simulink model "building_EXAMPLE_v1"  (R2016b)
settings: Solver=ode23tb  StartTime=-building.preruntime+8760*3600  StopTime=building.runtime+8760*3600  MaxStep=600  EnableMultiTasking=on
StartFcn:
  | tic
StopFcn:
  | toc
values from neighbouring files (symbols this model uses):
  building = create_building_automatic(building, modify, import_mode, name_XML, name_EXCEL, name_PHPP, NUMBEROFZONES)    [work_EXAMPLE_v1.m]
undefined symbols (not defined in the file or in its folder): A, B, C, cp, Dd, Dreifach, FluidMix, get_building, ID, MassFlow, p, Pressure, Qdot_C, Qdot_C_energy, Qdot_H, Qdot_H_energy, Qdot_I_electricity, Qdot_I_electricity_energy, Qdot_I_light, Qdot_I_light_energy, Qdot_I_person, Qdot_I_person_energy, Qdot_S, Qdot_S_energy, Qdot_T_ground, Qdot_T_ground_energy, Qdot_T_neighbour, Qdot_T_neighbour_energy, Qdot_T_opaque, Qdot_T_opaque_energy, Qdot_T_window, Qdot_T_window_energy, Qdot_V_infiltration, Qdot_V_infiltration_energy, Qdot_V_mech, Qdot_V_mech_energy, Qdot_V_window, Qdot_V_window_energy, rho, Tc, Temperature, Tr, Ts, Wärmeschutzglas, x_CO2, x_H2O, x_VOC
libraries: carnotUIBK x1931, carnot x83, simulink_extras x22, simulink x12
(part 35 of 35)

== system building_EXAMPLE_v1/HVAC pipes/ventilation_pipe_out_1/mix4 ==
  THB_1 : Inport
  THB_2 : Inport  Port=2
  Add{,1..3} (4 alike) : Sum
  Bus Assignment : BusAssignment  AssignedSignals=Temperature,MassFlow,Pressure,FluidMix
  Bus Selector : BusSelector  OutputSignals=Temperature,MassFlow,Pressure,FluidMix
  Bus Selector2 : BusSelector  OutputSignals=Temperature,MassFlow,Pressure,FluidMix
  Divide : Product  Inputs=*/
  Divide1 : Product  Inputs=*/
  Divide2 : Product  Inputs=*/
  Product{,1..5} (6 alike) : Product
  THB : Outport
  wires:
  Add/1 -> Divide/1  "theta"
  Product1/1 -> Add/2
  Product/1 -> Add/1
  THB_1/1 -> Bus Assignment/1, Bus Selector/1
  Add2/1 -> Divide1/1  "p"
  Product2/1 -> Add2/1
  Product3/1 -> Add2/2
  THB_2/1 -> Bus Selector2/1
  Product4/1 -> Add3/1
  Product5/1 -> Add3/2
  Add3/1 -> Divide2/1  "x"
  Add1/1 -> Divide/2, Divide1/2, Divide2/2, Bus Assignment/3  "massflow"
  Bus Assignment/1 -> THB/1
  Divide2/1 -> Bus Assignment/5
  Divide1/1 -> Bus Assignment/4
  Divide/1 -> Bus Assignment/2
  Bus Selector/1 -> Product/1  "<Temperature>"
  Bus Selector2/1 -> Product1/1  "<Temperature>"
  Bus Selector/3 -> Product2/2  "<Pressure>"
  Bus Selector2/3 -> Product3/2  "<Pressure>"
  Bus Selector/4 -> Product4/2  "<FluidMix>"
  Bus Selector2/4 -> Product5/2  "<FluidMix>"
  Bus Selector/2 -> Product4/1, Product2/1, Add1/1, Product/2  "<MassFlow>"
  Bus Selector2/2 -> Add1/2, Product1/2, Product5/1, Product3/1  "<MassFlow>"

== system building_EXAMPLE_v1/HVAC pipes/ventilation_pipe_out_1/mix5 ==
  THB_1 : Inport
  THB_2 : Inport  Port=2
  Add{,1..3} (4 alike) : Sum
  Bus Assignment : BusAssignment  AssignedSignals=Temperature,MassFlow,Pressure,FluidMix
  Bus Selector : BusSelector  OutputSignals=Temperature,MassFlow,Pressure,FluidMix
  Bus Selector2 : BusSelector  OutputSignals=Temperature,MassFlow,Pressure,FluidMix
  Divide : Product  Inputs=*/
  Divide1 : Product  Inputs=*/
  Divide2 : Product  Inputs=*/
  Product{,1..5} (6 alike) : Product
  THB : Outport
  wires:
  Bus Selector2/2 -> Product3/1, Product5/1, Product1/2, Add1/2  "<MassFlow>"
  Bus Selector/2 -> Product/2, Add1/1, Product2/1, Product4/1  "<MassFlow>"
  Bus Selector2/4 -> Product5/2  "<FluidMix>"
  Bus Selector/4 -> Product4/2  "<FluidMix>"
  Bus Selector2/3 -> Product3/2  "<Pressure>"
  Bus Selector/3 -> Product2/2  "<Pressure>"
  Bus Selector2/1 -> Product1/1  "<Temperature>"
  Bus Selector/1 -> Product/1  "<Temperature>"
  Divide/1 -> Bus Assignment/2
  Divide1/1 -> Bus Assignment/4
  Divide2/1 -> Bus Assignment/5
  Bus Assignment/1 -> THB/1
  Add1/1 -> Bus Assignment/3, Divide2/2, Divide1/2, Divide/2  "massflow"
  Add3/1 -> Divide2/1  "x"
  Product5/1 -> Add3/2
  Product4/1 -> Add3/1
  THB_2/1 -> Bus Selector2/1
  Product3/1 -> Add2/2
  Product2/1 -> Add2/1
  Add2/1 -> Divide1/1  "p"
  THB_1/1 -> Bus Selector/1, Bus Assignment/1
  Product/1 -> Add/1
  Product1/1 -> Add/2
  Add/1 -> Divide/1  "theta"

== system building_EXAMPLE_v1/HVAC pipes/ventilation_pipe_out_1/mix6 ==
  THB_1 : Inport
  THB_2 : Inport  Port=2
  Add{,1..3} (4 alike) : Sum
  Bus Assignment : BusAssignment  AssignedSignals=Temperature,MassFlow,Pressure,FluidMix
  Bus Selector : BusSelector  OutputSignals=Temperature,MassFlow,Pressure,FluidMix
  Bus Selector2 : BusSelector  OutputSignals=Temperature,MassFlow,Pressure,FluidMix
  Divide : Product  Inputs=*/
  Divide1 : Product  Inputs=*/
  Divide2 : Product  Inputs=*/
  Product{,1..5} (6 alike) : Product
  THB : Outport
  wires:
  Add/1 -> Divide/1  "theta"
  Product1/1 -> Add/2
  Product/1 -> Add/1
  THB_1/1 -> Bus Assignment/1, Bus Selector/1
  Add2/1 -> Divide1/1  "p"
  Product2/1 -> Add2/1
  Product3/1 -> Add2/2
  THB_2/1 -> Bus Selector2/1
  Product4/1 -> Add3/1
  Product5/1 -> Add3/2
  Add3/1 -> Divide2/1  "x"
  Add1/1 -> Divide/2, Divide1/2, Divide2/2, Bus Assignment/3  "massflow"
  Bus Assignment/1 -> THB/1
  Divide2/1 -> Bus Assignment/5
  Divide1/1 -> Bus Assignment/4
  Divide/1 -> Bus Assignment/2
  Bus Selector/1 -> Product/1  "<Temperature>"
  Bus Selector2/1 -> Product1/1  "<Temperature>"
  Bus Selector/3 -> Product2/2  "<Pressure>"
  Bus Selector2/3 -> Product3/2  "<Pressure>"
  Bus Selector/4 -> Product4/2  "<FluidMix>"
  Bus Selector2/4 -> Product5/2  "<FluidMix>"
  Bus Selector/2 -> Product4/1, Product2/1, Add1/1, Product/2  "<MassFlow>"
  Bus Selector2/2 -> Add1/2, Product1/2, Product5/1, Product3/1  "<MassFlow>"

== system building_EXAMPLE_v1/HVAC pipes/ventilation_pipe_out_1/mix7 ==
  THB_1 : Inport
  THB_2 : Inport  Port=2
  Add{,1..3} (4 alike) : Sum
  Bus Assignment : BusAssignment  AssignedSignals=Temperature,MassFlow,Pressure,FluidMix
  Bus Selector : BusSelector  OutputSignals=Temperature,MassFlow,Pressure,FluidMix
  Bus Selector2 : BusSelector  OutputSignals=Temperature,MassFlow,Pressure,FluidMix
  Divide : Product  Inputs=*/
  Divide1 : Product  Inputs=*/
  Divide2 : Product  Inputs=*/
  Product{,1..5} (6 alike) : Product
  THB : Outport
  wires:
  Bus Selector2/2 -> Product3/1, Product5/1, Product1/2, Add1/2  "<MassFlow>"
  Bus Selector/2 -> Product/2, Add1/1, Product2/1, Product4/1  "<MassFlow>"
  Bus Selector2/4 -> Product5/2  "<FluidMix>"
  Bus Selector/4 -> Product4/2  "<FluidMix>"
  Bus Selector2/3 -> Product3/2  "<Pressure>"
  Bus Selector/3 -> Product2/2  "<Pressure>"
  Bus Selector2/1 -> Product1/1  "<Temperature>"
  Bus Selector/1 -> Product/1  "<Temperature>"
  Divide/1 -> Bus Assignment/2
  Divide1/1 -> Bus Assignment/4
  Divide2/1 -> Bus Assignment/5
  Bus Assignment/1 -> THB/1
  Add1/1 -> Bus Assignment/3, Divide2/2, Divide1/2, Divide/2  "massflow"
  Add3/1 -> Divide2/1  "x"
  Product5/1 -> Add3/2
  Product4/1 -> Add3/1
  THB_2/1 -> Bus Selector2/1
  Product3/1 -> Add2/2
  Product2/1 -> Add2/1
  Add2/1 -> Divide1/1  "p"
  THB_1/1 -> Bus Selector/1, Bus Assignment/1
  Product/1 -> Add/1
  Product1/1 -> Add/2
  Add/1 -> Divide/1  "theta"

== system building_EXAMPLE_v1/HVAC pipes/ventilation_pipe_out_1/mix8 ==
  THB_1 : Inport
  THB_2 : Inport  Port=2
  Add{,1..3} (4 alike) : Sum
  Bus Assignment : BusAssignment  AssignedSignals=Temperature,MassFlow,Pressure,FluidMix
  Bus Selector : BusSelector  OutputSignals=Temperature,MassFlow,Pressure,FluidMix
  Bus Selector2 : BusSelector  OutputSignals=Temperature,MassFlow,Pressure,FluidMix
  Divide : Product  Inputs=*/
  Divide1 : Product  Inputs=*/
  Divide2 : Product  Inputs=*/
  Product{,1..5} (6 alike) : Product
  THB : Outport
  wires:
  Add/1 -> Divide/1  "theta"
  Product1/1 -> Add/2
  Product/1 -> Add/1
  THB_1/1 -> Bus Assignment/1, Bus Selector/1
  Add2/1 -> Divide1/1  "p"
  Product2/1 -> Add2/1
  Product3/1 -> Add2/2
  THB_2/1 -> Bus Selector2/1
  Product4/1 -> Add3/1
  Product5/1 -> Add3/2
  Add3/1 -> Divide2/1  "x"
  Add1/1 -> Divide/2, Divide1/2, Divide2/2, Bus Assignment/3  "massflow"
  Bus Assignment/1 -> THB/1
  Divide2/1 -> Bus Assignment/5
  Divide1/1 -> Bus Assignment/4
  Divide/1 -> Bus Assignment/2
  Bus Selector/1 -> Product/1  "<Temperature>"
  Bus Selector2/1 -> Product1/1  "<Temperature>"
  Bus Selector/3 -> Product2/2  "<Pressure>"
  Bus Selector2/3 -> Product3/2  "<Pressure>"
  Bus Selector/4 -> Product4/2  "<FluidMix>"
  Bus Selector2/4 -> Product5/2  "<FluidMix>"
  Bus Selector/2 -> Product4/1, Product2/1, Add1/1, Product/2  "<MassFlow>"
  Bus Selector2/2 -> Add1/2, Product1/2, Product5/1, Product3/1  "<MassFlow>"

== system building_EXAMPLE_v1/DATALOGGER/logger_BDB/z1/Subsystem ==
  In1 : Inport
  Integrator1 : Integrator
  Ws->kWh : Gain  Gain=1/3600/1000
  Out1 : Outport
  wires:
  Ws->kWh/1 -> Out1/1
  Integrator1/1 -> Ws->kWh/1
  In1/1 -> Integrator1/1

== system building_EXAMPLE_v1/DATALOGGER/logger_BDB/z1/Subsystem1 ==
  In1 : Inport
  Integrator1 : Integrator
  Ws->kWh : Gain  Gain=1/3600/1000
  Out1 : Outport
  wires:
  In1/1 -> Integrator1/1
  Integrator1/1 -> Ws->kWh/1
  Ws->kWh/1 -> Out1/1

== system building_EXAMPLE_v1/DATALOGGER/logger_BDB/z1/Subsystem10 ==
  In1 : Inport
  Integrator1 : Integrator
  Ws->kWh : Gain  Gain=1/3600/1000
  Out1 : Outport
  wires:
  Ws->kWh/1 -> Out1/1
  Integrator1/1 -> Ws->kWh/1
  In1/1 -> Integrator1/1

== system building_EXAMPLE_v1/DATALOGGER/logger_BDB/z1/Subsystem11 ==
  In1 : Inport
  Integrator1 : Integrator
  Ws->kWh : Gain  Gain=1/3600/1000
  Out1 : Outport
  wires:
  In1/1 -> Integrator1/1
  Integrator1/1 -> Ws->kWh/1
  Ws->kWh/1 -> Out1/1

== system building_EXAMPLE_v1/DATALOGGER/logger_BDB/z1/Subsystem12 ==
  In1 : Inport
  Integrator1 : Integrator
  Ws->kWh : Gain  Gain=1/3600/1000
  Out1 : Outport
  wires:
  Ws->kWh/1 -> Out1/1
  Integrator1/1 -> Ws->kWh/1
  In1/1 -> Integrator1/1

== system building_EXAMPLE_v1/DATALOGGER/logger_BDB/z1/Subsystem2 ==
  In1 : Inport
  Integrator1 : Integrator
  Ws->kWh : Gain  Gain=1/3600/1000
  Out1 : Outport
  wires:
  Ws->kWh/1 -> Out1/1
  Integrator1/1 -> Ws->kWh/1
  In1/1 -> Integrator1/1

== system building_EXAMPLE_v1/DATALOGGER/logger_BDB/z1/Subsystem3 ==
  In1 : Inport
  Integrator1 : Integrator
  Ws->kWh : Gain  Gain=1/3600/1000
  Out1 : Outport
  wires:
  In1/1 -> Integrator1/1
  Integrator1/1 -> Ws->kWh/1
  Ws->kWh/1 -> Out1/1

== system building_EXAMPLE_v1/DATALOGGER/logger_BDB/z1/Subsystem4 ==
  In1 : Inport
  Integrator1 : Integrator
  Ws->kWh : Gain  Gain=1/3600/1000
  Out1 : Outport
  wires:
  Ws->kWh/1 -> Out1/1
  Integrator1/1 -> Ws->kWh/1
  In1/1 -> Integrator1/1

== system building_EXAMPLE_v1/DATALOGGER/logger_BDB/z1/Subsystem5 ==
  In1 : Inport
  Integrator1 : Integrator
  Ws->kWh : Gain  Gain=1/3600/1000
  Out1 : Outport
  wires:
  In1/1 -> Integrator1/1
  Integrator1/1 -> Ws->kWh/1
  Ws->kWh/1 -> Out1/1

== system building_EXAMPLE_v1/DATALOGGER/logger_BDB/z1/Subsystem6 ==
  In1 : Inport
  Integrator1 : Integrator
  Ws->kWh : Gain  Gain=1/3600/1000
  Out1 : Outport
  wires:
  Ws->kWh/1 -> Out1/1
  Integrator1/1 -> Ws->kWh/1
  In1/1 -> Integrator1/1

== system building_EXAMPLE_v1/DATALOGGER/logger_BDB/z1/Subsystem7 ==
  In1 : Inport
  Integrator1 : Integrator
  Ws->kWh : Gain  Gain=1/3600/1000
  Out1 : Outport
  wires:
  In1/1 -> Integrator1/1
  Integrator1/1 -> Ws->kWh/1
  Ws->kWh/1 -> Out1/1

== system building_EXAMPLE_v1/DATALOGGER/logger_BDB/z1/Subsystem8 ==
  In1 : Inport
  Integrator1 : Integrator
  Ws->kWh : Gain  Gain=1/3600/1000
  Out1 : Outport
  wires:
  Ws->kWh/1 -> Out1/1
  Integrator1/1 -> Ws->kWh/1
  In1/1 -> Integrator1/1

== system building_EXAMPLE_v1/DATALOGGER/logger_BDB/z1/Subsystem9 ==
  In1 : Inport
  Integrator1 : Integrator
  Ws->kWh : Gain  Gain=1/3600/1000
  Out1 : Outport
  wires:
  In1/1 -> Integrator1/1
  Integrator1/1 -> Ws->kWh/1
  Ws->kWh/1 -> Out1/1

== system building_EXAMPLE_v1/DATALOGGER/logger_BDB/z10/Subsystem ==
  In1 : Inport
  Integrator1 : Integrator
  Ws->kWh : Gain  Gain=1/3600/1000
  Out1 : Outport
  wires:
  In1/1 -> Integrator1/1
  Integrator1/1 -> Ws->kWh/1
  Ws->kWh/1 -> Out1/1

== system building_EXAMPLE_v1/DATALOGGER/logger_BDB/z10/Subsystem1 ==
  In1 : Inport
  Integrator1 : Integrator
  Ws->kWh : Gain  Gain=1/3600/1000
  Out1 : Outport
  wires:
  Ws->kWh/1 -> Out1/1
  Integrator1/1 -> Ws->kWh/1
  In1/1 -> Integrator1/1

== system building_EXAMPLE_v1/DATALOGGER/logger_BDB/z10/Subsystem10 ==
  In1 : Inport
  Integrator1 : Integrator
  Ws->kWh : Gain  Gain=1/3600/1000
  Out1 : Outport
  wires:
  In1/1 -> Integrator1/1
  Integrator1/1 -> Ws->kWh/1
  Ws->kWh/1 -> Out1/1

== system building_EXAMPLE_v1/DATALOGGER/logger_BDB/z10/Subsystem11 ==
  In1 : Inport
  Integrator1 : Integrator
  Ws->kWh : Gain  Gain=1/3600/1000
  Out1 : Outport
  wires:
  Ws->kWh/1 -> Out1/1
  Integrator1/1 -> Ws->kWh/1
  In1/1 -> Integrator1/1

== system building_EXAMPLE_v1/DATALOGGER/logger_BDB/z10/Subsystem12 ==
  In1 : Inport
  Integrator1 : Integrator
  Ws->kWh : Gain  Gain=1/3600/1000
  Out1 : Outport
  wires:
  In1/1 -> Integrator1/1
  Integrator1/1 -> Ws->kWh/1
  Ws->kWh/1 -> Out1/1

== system building_EXAMPLE_v1/DATALOGGER/logger_BDB/z10/Subsystem2 ==
  In1 : Inport
  Integrator1 : Integrator
  Ws->kWh : Gain  Gain=1/3600/1000
  Out1 : Outport
  wires:
  In1/1 -> Integrator1/1
  Integrator1/1 -> Ws->kWh/1
  Ws->kWh/1 -> Out1/1

== system building_EXAMPLE_v1/DATALOGGER/logger_BDB/z10/Subsystem3 ==
  In1 : Inport
  Integrator1 : Integrator
  Ws->kWh : Gain  Gain=1/3600/1000
  Out1 : Outport
  wires:
  Ws->kWh/1 -> Out1/1
  Integrator1/1 -> Ws->kWh/1
  In1/1 -> Integrator1/1

== system building_EXAMPLE_v1/DATALOGGER/logger_BDB/z10/Subsystem4 ==
  In1 : Inport
  Integrator1 : Integrator
  Ws->kWh : Gain  Gain=1/3600/1000
  Out1 : Outport
  wires:
  In1/1 -> Integrator1/1
  Integrator1/1 -> Ws->kWh/1
  Ws->kWh/1 -> Out1/1

== system building_EXAMPLE_v1/DATALOGGER/logger_BDB/z10/Subsystem5 ==
  In1 : Inport
  Integrator1 : Integrator
  Ws->kWh : Gain  Gain=1/3600/1000
  Out1 : Outport
  wires:
  Ws->kWh/1 -> Out1/1
  Integrator1/1 -> Ws->kWh/1
  In1/1 -> Integrator1/1

== system building_EXAMPLE_v1/DATALOGGER/logger_BDB/z10/Subsystem6 ==
  In1 : Inport
  Integrator1 : Integrator
  Ws->kWh : Gain  Gain=1/3600/1000
  Out1 : Outport
  wires:
  In1/1 -> Integrator1/1
  Integrator1/1 -> Ws->kWh/1
  Ws->kWh/1 -> Out1/1

== system building_EXAMPLE_v1/DATALOGGER/logger_BDB/z10/Subsystem7 ==
  In1 : Inport
  Integrator1 : Integrator
  Ws->kWh : Gain  Gain=1/3600/1000
  Out1 : Outport
  wires:
  Ws->kWh/1 -> Out1/1
  Integrator1/1 -> Ws->kWh/1
  In1/1 -> Integrator1/1

== system building_EXAMPLE_v1/DATALOGGER/logger_BDB/z10/Subsystem8 ==
  In1 : Inport
  Integrator1 : Integrator
  Ws->kWh : Gain  Gain=1/3600/1000
  Out1 : Outport
  wires:
  In1/1 -> Integrator1/1
  Integrator1/1 -> Ws->kWh/1
  Ws->kWh/1 -> Out1/1

== system building_EXAMPLE_v1/DATALOGGER/logger_BDB/z10/Subsystem9 ==
  In1 : Inport
  Integrator1 : Integrator
  Ws->kWh : Gain  Gain=1/3600/1000
  Out1 : Outport
  wires:
  Ws->kWh/1 -> Out1/1
  Integrator1/1 -> Ws->kWh/1
  In1/1 -> Integrator1/1

== system building_EXAMPLE_v1/DATALOGGER/logger_BDB/z2/Subsystem ==
  In1 : Inport
  Integrator1 : Integrator
  Ws->kWh : Gain  Gain=1/3600/1000
  Out1 : Outport
  wires:
  In1/1 -> Integrator1/1
  Integrator1/1 -> Ws->kWh/1
  Ws->kWh/1 -> Out1/1

== system building_EXAMPLE_v1/DATALOGGER/logger_BDB/z2/Subsystem1 ==
  In1 : Inport
  Integrator1 : Integrator
  Ws->kWh : Gain  Gain=1/3600/1000
  Out1 : Outport
  wires:
  Ws->kWh/1 -> Out1/1
  Integrator1/1 -> Ws->kWh/1
  In1/1 -> Integrator1/1

== system building_EXAMPLE_v1/DATALOGGER/logger_BDB/z2/Subsystem10 ==
  In1 : Inport
  Integrator1 : Integrator
  Ws->kWh : Gain  Gain=1/3600/1000
  Out1 : Outport
  wires:
  In1/1 -> Integrator1/1
  Integrator1/1 -> Ws->kWh/1
  Ws->kWh/1 -> Out1/1

== system building_EXAMPLE_v1/DATALOGGER/logger_BDB/z2/Subsystem11 ==
  In1 : Inport
  Integrator1 : Integrator
  Ws->kWh : Gain  Gain=1/3600/1000
  Out1 : Outport
  wires:
  Ws->kWh/1 -> Out1/1
  Integrator1/1 -> Ws->kWh/1
  In1/1 -> Integrator1/1

== system building_EXAMPLE_v1/DATALOGGER/logger_BDB/z2/Subsystem12 ==
  In1 : Inport
  Integrator1 : Integrator
  Ws->kWh : Gain  Gain=1/3600/1000
  Out1 : Outport
  wires:
  In1/1 -> Integrator1/1
  Integrator1/1 -> Ws->kWh/1
  Ws->kWh/1 -> Out1/1

== system building_EXAMPLE_v1/DATALOGGER/logger_BDB/z2/Subsystem2 ==
  In1 : Inport
  Integrator1 : Integrator
  Ws->kWh : Gain  Gain=1/3600/1000
  Out1 : Outport
  wires:
  In1/1 -> Integrator1/1
  Integrator1/1 -> Ws->kWh/1
  Ws->kWh/1 -> Out1/1

== system building_EXAMPLE_v1/DATALOGGER/logger_BDB/z2/Subsystem3 ==
  In1 : Inport
  Integrator1 : Integrator
  Ws->kWh : Gain  Gain=1/3600/1000
  Out1 : Outport
  wires:
  Ws->kWh/1 -> Out1/1
  Integrator1/1 -> Ws->kWh/1
  In1/1 -> Integrator1/1

== system building_EXAMPLE_v1/DATALOGGER/logger_BDB/z2/Subsystem4 ==
  In1 : Inport
  Integrator1 : Integrator
  Ws->kWh : Gain  Gain=1/3600/1000
  Out1 : Outport
  wires:
  In1/1 -> Integrator1/1
  Integrator1/1 -> Ws->kWh/1
  Ws->kWh/1 -> Out1/1

== system building_EXAMPLE_v1/DATALOGGER/logger_BDB/z2/Subsystem5 ==
  In1 : Inport
  Integrator1 : Integrator
  Ws->kWh : Gain  Gain=1/3600/1000
  Out1 : Outport
  wires:
  Ws->kWh/1 -> Out1/1
  Integrator1/1 -> Ws->kWh/1
  In1/1 -> Integrator1/1

== system building_EXAMPLE_v1/DATALOGGER/logger_BDB/z2/Subsystem6 ==
  In1 : Inport
  Integrator1 : Integrator
  Ws->kWh : Gain  Gain=1/3600/1000
  Out1 : Outport
  wires:
  In1/1 -> Integrator1/1
  Integrator1/1 -> Ws->kWh/1
  Ws->kWh/1 -> Out1/1

== system building_EXAMPLE_v1/DATALOGGER/logger_BDB/z2/Subsystem7 ==
  In1 : Inport
  Integrator1 : Integrator
  Ws->kWh : Gain  Gain=1/3600/1000
  Out1 : Outport
  wires:
  Ws->kWh/1 -> Out1/1
  Integrator1/1 -> Ws->kWh/1
  In1/1 -> Integrator1/1

== system building_EXAMPLE_v1/DATALOGGER/logger_BDB/z2/Subsystem8 ==
  In1 : Inport
  Integrator1 : Integrator
  Ws->kWh : Gain  Gain=1/3600/1000
  Out1 : Outport
  wires:
  In1/1 -> Integrator1/1
  Integrator1/1 -> Ws->kWh/1
  Ws->kWh/1 -> Out1/1

== system building_EXAMPLE_v1/DATALOGGER/logger_BDB/z2/Subsystem9 ==
  In1 : Inport
  Integrator1 : Integrator
  Ws->kWh : Gain  Gain=1/3600/1000
  Out1 : Outport
  wires:
  Ws->kWh/1 -> Out1/1
  Integrator1/1 -> Ws->kWh/1
  In1/1 -> Integrator1/1

== system building_EXAMPLE_v1/DATALOGGER/logger_BDB/z3/Subsystem ==
  In1 : Inport
  Integrator1 : Integrator
  Ws->kWh : Gain  Gain=1/3600/1000
  Out1 : Outport
  wires:
  Ws->kWh/1 -> Out1/1
  Integrator1/1 -> Ws->kWh/1
  In1/1 -> Integrator1/1

== system building_EXAMPLE_v1/DATALOGGER/logger_BDB/z3/Subsystem1 ==
  In1 : Inport
  Integrator1 : Integrator
  Ws->kWh : Gain  Gain=1/3600/1000
  Out1 : Outport
  wires:
  In1/1 -> Integrator1/1
  Integrator1/1 -> Ws->kWh/1
  Ws->kWh/1 -> Out1/1

== system building_EXAMPLE_v1/DATALOGGER/logger_BDB/z3/Subsystem10 ==
  In1 : Inport
  Integrator1 : Integrator
  Ws->kWh : Gain  Gain=1/3600/1000
  Out1 : Outport
  wires:
  Ws->kWh/1 -> Out1/1
  Integrator1/1 -> Ws->kWh/1
  In1/1 -> Integrator1/1

== system building_EXAMPLE_v1/DATALOGGER/logger_BDB/z3/Subsystem11 ==
  In1 : Inport
  Integrator1 : Integrator
  Ws->kWh : Gain  Gain=1/3600/1000
  Out1 : Outport
  wires:
  In1/1 -> Integrator1/1
  Integrator1/1 -> Ws->kWh/1
  Ws->kWh/1 -> Out1/1

== system building_EXAMPLE_v1/DATALOGGER/logger_BDB/z3/Subsystem12 ==
  In1 : Inport
  Integrator1 : Integrator
  Ws->kWh : Gain  Gain=1/3600/1000
  Out1 : Outport
  wires:
  Ws->kWh/1 -> Out1/1
  Integrator1/1 -> Ws->kWh/1
  In1/1 -> Integrator1/1

== system building_EXAMPLE_v1/DATALOGGER/logger_BDB/z3/Subsystem2 ==
  In1 : Inport
  Integrator1 : Integrator
  Ws->kWh : Gain  Gain=1/3600/1000
  Out1 : Outport
  wires:
  Ws->kWh/1 -> Out1/1
  Integrator1/1 -> Ws->kWh/1
  In1/1 -> Integrator1/1

== system building_EXAMPLE_v1/DATALOGGER/logger_BDB/z3/Subsystem3 ==
  In1 : Inport
  Integrator1 : Integrator
  Ws->kWh : Gain  Gain=1/3600/1000
  Out1 : Outport
  wires:
  In1/1 -> Integrator1/1
  Integrator1/1 -> Ws->kWh/1
  Ws->kWh/1 -> Out1/1

== system building_EXAMPLE_v1/DATALOGGER/logger_BDB/z3/Subsystem4 ==
  In1 : Inport
  Integrator1 : Integrator
  Ws->kWh : Gain  Gain=1/3600/1000
  Out1 : Outport
  wires:
  Ws->kWh/1 -> Out1/1
  Integrator1/1 -> Ws->kWh/1
  In1/1 -> Integrator1/1

== system building_EXAMPLE_v1/DATALOGGER/logger_BDB/z3/Subsystem5 ==
  In1 : Inport
  Integrator1 : Integrator
  Ws->kWh : Gain  Gain=1/3600/1000
  Out1 : Outport
  wires:
  In1/1 -> Integrator1/1
  Integrator1/1 -> Ws->kWh/1
  Ws->kWh/1 -> Out1/1

== system building_EXAMPLE_v1/DATALOGGER/logger_BDB/z3/Subsystem6 ==
  In1 : Inport
  Integrator1 : Integrator
  Ws->kWh : Gain  Gain=1/3600/1000
  Out1 : Outport
  wires:
  Ws->kWh/1 -> Out1/1
  Integrator1/1 -> Ws->kWh/1
  In1/1 -> Integrator1/1

== system building_EXAMPLE_v1/DATALOGGER/logger_BDB/z3/Subsystem7 ==
  In1 : Inport
  Integrator1 : Integrator
  Ws->kWh : Gain  Gain=1/3600/1000
  Out1 : Outport
  wires:
  In1/1 -> Integrator1/1
  Integrator1/1 -> Ws->kWh/1
  Ws->kWh/1 -> Out1/1

== system building_EXAMPLE_v1/DATALOGGER/logger_BDB/z3/Subsystem8 ==
  In1 : Inport
  Integrator1 : Integrator
  Ws->kWh : Gain  Gain=1/3600/1000
  Out1 : Outport
  wires:
  Ws->kWh/1 -> Out1/1
  Integrator1/1 -> Ws->kWh/1
  In1/1 -> Integrator1/1

== system building_EXAMPLE_v1/DATALOGGER/logger_BDB/z3/Subsystem9 ==
  In1 : Inport
  Integrator1 : Integrator
  Ws->kWh : Gain  Gain=1/3600/1000
  Out1 : Outport
  wires:
  In1/1 -> Integrator1/1
  Integrator1/1 -> Ws->kWh/1
  Ws->kWh/1 -> Out1/1

== system building_EXAMPLE_v1/DATALOGGER/logger_BDB/z4/Subsystem ==
  In1 : Inport
  Integrator1 : Integrator
  Ws->kWh : Gain  Gain=1/3600/1000
  Out1 : Outport
  wires:
  In1/1 -> Integrator1/1
  Integrator1/1 -> Ws->kWh/1
  Ws->kWh/1 -> Out1/1

== system building_EXAMPLE_v1/DATALOGGER/logger_BDB/z4/Subsystem1 ==
  In1 : Inport
  Integrator1 : Integrator
  Ws->kWh : Gain  Gain=1/3600/1000
  Out1 : Outport
  wires:
  Ws->kWh/1 -> Out1/1
  Integrator1/1 -> Ws->kWh/1
  In1/1 -> Integrator1/1

== system building_EXAMPLE_v1/DATALOGGER/logger_BDB/z4/Subsystem10 ==
  In1 : Inport
  Integrator1 : Integrator
  Ws->kWh : Gain  Gain=1/3600/1000
  Out1 : Outport
  wires:
  In1/1 -> Integrator1/1
  Integrator1/1 -> Ws->kWh/1
  Ws->kWh/1 -> Out1/1

== system building_EXAMPLE_v1/DATALOGGER/logger_BDB/z4/Subsystem11 ==
  In1 : Inport
  Integrator1 : Integrator
  Ws->kWh : Gain  Gain=1/3600/1000
  Out1 : Outport
  wires:
  Ws->kWh/1 -> Out1/1
  Integrator1/1 -> Ws->kWh/1
  In1/1 -> Integrator1/1

== system building_EXAMPLE_v1/DATALOGGER/logger_BDB/z4/Subsystem12 ==
  In1 : Inport
  Integrator1 : Integrator
  Ws->kWh : Gain  Gain=1/3600/1000
  Out1 : Outport
  wires:
  In1/1 -> Integrator1/1
  Integrator1/1 -> Ws->kWh/1
  Ws->kWh/1 -> Out1/1

== system building_EXAMPLE_v1/DATALOGGER/logger_BDB/z4/Subsystem2 ==
  In1 : Inport
  Integrator1 : Integrator
  Ws->kWh : Gain  Gain=1/3600/1000
  Out1 : Outport
  wires:
  In1/1 -> Integrator1/1
  Integrator1/1 -> Ws->kWh/1
  Ws->kWh/1 -> Out1/1

== system building_EXAMPLE_v1/DATALOGGER/logger_BDB/z4/Subsystem3 ==
  In1 : Inport
  Integrator1 : Integrator
  Ws->kWh : Gain  Gain=1/3600/1000
  Out1 : Outport
  wires:
  Ws->kWh/1 -> Out1/1
  Integrator1/1 -> Ws->kWh/1
  In1/1 -> Integrator1/1

== system building_EXAMPLE_v1/DATALOGGER/logger_BDB/z4/Subsystem4 ==
  In1 : Inport
  Integrator1 : Integrator
  Ws->kWh : Gain  Gain=1/3600/1000
  Out1 : Outport
  wires:
  In1/1 -> Integrator1/1
  Integrator1/1 -> Ws->kWh/1
  Ws->kWh/1 -> Out1/1

== system building_EXAMPLE_v1/DATALOGGER/logger_BDB/z4/Subsystem5 ==
  In1 : Inport
  Integrator1 : Integrator
  Ws->kWh : Gain  Gain=1/3600/1000
  Out1 : Outport
  wires:
  Ws->kWh/1 -> Out1/1
  Integrator1/1 -> Ws->kWh/1
  In1/1 -> Integrator1/1

== system building_EXAMPLE_v1/DATALOGGER/logger_BDB/z4/Subsystem6 ==
  In1 : Inport
  Integrator1 : Integrator
  Ws->kWh : Gain  Gain=1/3600/1000
  Out1 : Outport
  wires:
  In1/1 -> Integrator1/1
  Integrator1/1 -> Ws->kWh/1
  Ws->kWh/1 -> Out1/1

== system building_EXAMPLE_v1/DATALOGGER/logger_BDB/z4/Subsystem7 ==
  In1 : Inport
  Integrator1 : Integrator
  Ws->kWh : Gain  Gain=1/3600/1000
  Out1 : Outport
  wires:
  Ws->kWh/1 -> Out1/1
  Integrator1/1 -> Ws->kWh/1
  In1/1 -> Integrator1/1

== system building_EXAMPLE_v1/DATALOGGER/logger_BDB/z4/Subsystem8 ==
  In1 : Inport
  Integrator1 : Integrator
  Ws->kWh : Gain  Gain=1/3600/1000
  Out1 : Outport
  wires:
  In1/1 -> Integrator1/1
  Integrator1/1 -> Ws->kWh/1
  Ws->kWh/1 -> Out1/1

== system building_EXAMPLE_v1/DATALOGGER/logger_BDB/z4/Subsystem9 ==
  In1 : Inport
  Integrator1 : Integrator
  Ws->kWh : Gain  Gain=1/3600/1000
  Out1 : Outport
  wires:
  Ws->kWh/1 -> Out1/1
  Integrator1/1 -> Ws->kWh/1
  In1/1 -> Integrator1/1

== system building_EXAMPLE_v1/DATALOGGER/logger_BDB/z5/Subsystem ==
  In1 : Inport
  Integrator1 : Integrator
  Ws->kWh : Gain  Gain=1/3600/1000
  Out1 : Outport
  wires:
  Ws->kWh/1 -> Out1/1
  Integrator1/1 -> Ws->kWh/1
  In1/1 -> Integrator1/1

== system building_EXAMPLE_v1/DATALOGGER/logger_BDB/z5/Subsystem1 ==
  In1 : Inport
  Integrator1 : Integrator
  Ws->kWh : Gain  Gain=1/3600/1000
  Out1 : Outport
  wires:
  In1/1 -> Integrator1/1
  Integrator1/1 -> Ws->kWh/1
  Ws->kWh/1 -> Out1/1

== system building_EXAMPLE_v1/DATALOGGER/logger_BDB/z5/Subsystem10 ==
  In1 : Inport
  Integrator1 : Integrator
  Ws->kWh : Gain  Gain=1/3600/1000
  Out1 : Outport
  wires:
  Ws->kWh/1 -> Out1/1
  Integrator1/1 -> Ws->kWh/1
  In1/1 -> Integrator1/1

== system building_EXAMPLE_v1/DATALOGGER/logger_BDB/z5/Subsystem11 ==
  In1 : Inport
  Integrator1 : Integrator
  Ws->kWh : Gain  Gain=1/3600/1000
  Out1 : Outport
  wires:
  In1/1 -> Integrator1/1
  Integrator1/1 -> Ws->kWh/1
  Ws->kWh/1 -> Out1/1

== system building_EXAMPLE_v1/DATALOGGER/logger_BDB/z5/Subsystem12 ==
  In1 : Inport
  Integrator1 : Integrator
  Ws->kWh : Gain  Gain=1/3600/1000
  Out1 : Outport
  wires:
  Ws->kWh/1 -> Out1/1
  Integrator1/1 -> Ws->kWh/1
  In1/1 -> Integrator1/1

== system building_EXAMPLE_v1/DATALOGGER/logger_BDB/z5/Subsystem2 ==
  In1 : Inport
  Integrator1 : Integrator
  Ws->kWh : Gain  Gain=1/3600/1000
  Out1 : Outport
  wires:
  Ws->kWh/1 -> Out1/1
  Integrator1/1 -> Ws->kWh/1
  In1/1 -> Integrator1/1

== system building_EXAMPLE_v1/DATALOGGER/logger_BDB/z5/Subsystem3 ==
  In1 : Inport
  Integrator1 : Integrator
  Ws->kWh : Gain  Gain=1/3600/1000
  Out1 : Outport
  wires:
  In1/1 -> Integrator1/1
  Integrator1/1 -> Ws->kWh/1
  Ws->kWh/1 -> Out1/1

== system building_EXAMPLE_v1/DATALOGGER/logger_BDB/z5/Subsystem4 ==
  In1 : Inport
  Integrator1 : Integrator
  Ws->kWh : Gain  Gain=1/3600/1000
  Out1 : Outport
  wires:
  Ws->kWh/1 -> Out1/1
  Integrator1/1 -> Ws->kWh/1
  In1/1 -> Integrator1/1

== system building_EXAMPLE_v1/DATALOGGER/logger_BDB/z5/Subsystem5 ==
  In1 : Inport
  Integrator1 : Integrator
  Ws->kWh : Gain  Gain=1/3600/1000
  Out1 : Outport
  wires:
  In1/1 -> Integrator1/1
  Integrator1/1 -> Ws->kWh/1
  Ws->kWh/1 -> Out1/1

== system building_EXAMPLE_v1/DATALOGGER/logger_BDB/z5/Subsystem6 ==
  In1 : Inport
  Integrator1 : Integrator
  Ws->kWh : Gain  Gain=1/3600/1000
  Out1 : Outport
  wires:
  Ws->kWh/1 -> Out1/1
  Integrator1/1 -> Ws->kWh/1
  In1/1 -> Integrator1/1

== system building_EXAMPLE_v1/DATALOGGER/logger_BDB/z5/Subsystem7 ==
  In1 : Inport
  Integrator1 : Integrator
  Ws->kWh : Gain  Gain=1/3600/1000
  Out1 : Outport
  wires:
  In1/1 -> Integrator1/1
  Integrator1/1 -> Ws->kWh/1
  Ws->kWh/1 -> Out1/1

== system building_EXAMPLE_v1/DATALOGGER/logger_BDB/z5/Subsystem8 ==
  In1 : Inport
  Integrator1 : Integrator
  Ws->kWh : Gain  Gain=1/3600/1000
  Out1 : Outport
  wires:
  Ws->kWh/1 -> Out1/1
  Integrator1/1 -> Ws->kWh/1
  In1/1 -> Integrator1/1

== system building_EXAMPLE_v1/DATALOGGER/logger_BDB/z5/Subsystem9 ==
  In1 : Inport
  Integrator1 : Integrator
  Ws->kWh : Gain  Gain=1/3600/1000
  Out1 : Outport
  wires:
  In1/1 -> Integrator1/1
  Integrator1/1 -> Ws->kWh/1
  Ws->kWh/1 -> Out1/1

== system building_EXAMPLE_v1/DATALOGGER/logger_BDB/z6/Subsystem ==
  In1 : Inport
  Integrator1 : Integrator
  Ws->kWh : Gain  Gain=1/3600/1000
  Out1 : Outport
  wires:
  In1/1 -> Integrator1/1
  Integrator1/1 -> Ws->kWh/1
  Ws->kWh/1 -> Out1/1

== system building_EXAMPLE_v1/DATALOGGER/logger_BDB/z6/Subsystem1 ==
  In1 : Inport
  Integrator1 : Integrator
  Ws->kWh : Gain  Gain=1/3600/1000
  Out1 : Outport
  wires:
  Ws->kWh/1 -> Out1/1
  Integrator1/1 -> Ws->kWh/1
  In1/1 -> Integrator1/1

== system building_EXAMPLE_v1/DATALOGGER/logger_BDB/z6/Subsystem10 ==
  In1 : Inport
  Integrator1 : Integrator
  Ws->kWh : Gain  Gain=1/3600/1000
  Out1 : Outport
  wires:
  In1/1 -> Integrator1/1
  Integrator1/1 -> Ws->kWh/1
  Ws->kWh/1 -> Out1/1

== system building_EXAMPLE_v1/DATALOGGER/logger_BDB/z6/Subsystem11 ==
  In1 : Inport
  Integrator1 : Integrator
  Ws->kWh : Gain  Gain=1/3600/1000
  Out1 : Outport
  wires:
  Ws->kWh/1 -> Out1/1
  Integrator1/1 -> Ws->kWh/1
  In1/1 -> Integrator1/1

== system building_EXAMPLE_v1/DATALOGGER/logger_BDB/z6/Subsystem12 ==
  In1 : Inport
  Integrator1 : Integrator
  Ws->kWh : Gain  Gain=1/3600/1000
  Out1 : Outport
  wires:
  In1/1 -> Integrator1/1
  Integrator1/1 -> Ws->kWh/1
  Ws->kWh/1 -> Out1/1

== system building_EXAMPLE_v1/DATALOGGER/logger_BDB/z6/Subsystem2 ==
  In1 : Inport
  Integrator1 : Integrator
  Ws->kWh : Gain  Gain=1/3600/1000
  Out1 : Outport
  wires:
  In1/1 -> Integrator1/1
  Integrator1/1 -> Ws->kWh/1
  Ws->kWh/1 -> Out1/1

== system building_EXAMPLE_v1/DATALOGGER/logger_BDB/z6/Subsystem3 ==
  In1 : Inport
  Integrator1 : Integrator
  Ws->kWh : Gain  Gain=1/3600/1000
  Out1 : Outport
  wires:
  Ws->kWh/1 -> Out1/1
  Integrator1/1 -> Ws->kWh/1
  In1/1 -> Integrator1/1

== system building_EXAMPLE_v1/DATALOGGER/logger_BDB/z6/Subsystem4 ==
  In1 : Inport
  Integrator1 : Integrator
  Ws->kWh : Gain  Gain=1/3600/1000
  Out1 : Outport
  wires:
  In1/1 -> Integrator1/1
  Integrator1/1 -> Ws->kWh/1
  Ws->kWh/1 -> Out1/1

== system building_EXAMPLE_v1/DATALOGGER/logger_BDB/z6/Subsystem5 ==
  In1 : Inport
  Integrator1 : Integrator
  Ws->kWh : Gain  Gain=1/3600/1000
  Out1 : Outport
  wires:
  Ws->kWh/1 -> Out1/1
  Integrator1/1 -> Ws->kWh/1
  In1/1 -> Integrator1/1

== system building_EXAMPLE_v1/DATALOGGER/logger_BDB/z6/Subsystem6 ==
  In1 : Inport
  Integrator1 : Integrator
  Ws->kWh : Gain  Gain=1/3600/1000
  Out1 : Outport
  wires:
  In1/1 -> Integrator1/1
  Integrator1/1 -> Ws->kWh/1
  Ws->kWh/1 -> Out1/1

== system building_EXAMPLE_v1/DATALOGGER/logger_BDB/z6/Subsystem7 ==
  In1 : Inport
  Integrator1 : Integrator
  Ws->kWh : Gain  Gain=1/3600/1000
  Out1 : Outport
  wires:
  Ws->kWh/1 -> Out1/1
  Integrator1/1 -> Ws->kWh/1
  In1/1 -> Integrator1/1

== system building_EXAMPLE_v1/DATALOGGER/logger_BDB/z6/Subsystem8 ==
  In1 : Inport
  Integrator1 : Integrator
  Ws->kWh : Gain  Gain=1/3600/1000
  Out1 : Outport
  wires:
  In1/1 -> Integrator1/1
  Integrator1/1 -> Ws->kWh/1
  Ws->kWh/1 -> Out1/1

== system building_EXAMPLE_v1/DATALOGGER/logger_BDB/z6/Subsystem9 ==
  In1 : Inport
  Integrator1 : Integrator
  Ws->kWh : Gain  Gain=1/3600/1000
  Out1 : Outport
  wires:
  Ws->kWh/1 -> Out1/1
  Integrator1/1 -> Ws->kWh/1
  In1/1 -> Integrator1/1

== system building_EXAMPLE_v1/DATALOGGER/logger_BDB/z7/Subsystem ==
  In1 : Inport
  Integrator1 : Integrator
  Ws->kWh : Gain  Gain=1/3600/1000
  Out1 : Outport
  wires:
  Ws->kWh/1 -> Out1/1
  Integrator1/1 -> Ws->kWh/1
  In1/1 -> Integrator1/1

== system building_EXAMPLE_v1/DATALOGGER/logger_BDB/z7/Subsystem1 ==
  In1 : Inport
  Integrator1 : Integrator
  Ws->kWh : Gain  Gain=1/3600/1000
  Out1 : Outport
  wires:
  In1/1 -> Integrator1/1
  Integrator1/1 -> Ws->kWh/1
  Ws->kWh/1 -> Out1/1

== system building_EXAMPLE_v1/DATALOGGER/logger_BDB/z7/Subsystem10 ==
  In1 : Inport
  Integrator1 : Integrator
  Ws->kWh : Gain  Gain=1/3600/1000
  Out1 : Outport
  wires:
  Ws->kWh/1 -> Out1/1
  Integrator1/1 -> Ws->kWh/1
  In1/1 -> Integrator1/1

== system building_EXAMPLE_v1/DATALOGGER/logger_BDB/z7/Subsystem11 ==
  In1 : Inport
  Integrator1 : Integrator
  Ws->kWh : Gain  Gain=1/3600/1000
  Out1 : Outport
  wires:
  In1/1 -> Integrator1/1
  Integrator1/1 -> Ws->kWh/1
  Ws->kWh/1 -> Out1/1

== system building_EXAMPLE_v1/DATALOGGER/logger_BDB/z7/Subsystem12 ==
  In1 : Inport
  Integrator1 : Integrator
  Ws->kWh : Gain  Gain=1/3600/1000
  Out1 : Outport
  wires:
  Ws->kWh/1 -> Out1/1
  Integrator1/1 -> Ws->kWh/1
  In1/1 -> Integrator1/1

== system building_EXAMPLE_v1/DATALOGGER/logger_BDB/z7/Subsystem2 ==
  In1 : Inport
  Integrator1 : Integrator
  Ws->kWh : Gain  Gain=1/3600/1000
  Out1 : Outport
  wires:
  Ws->kWh/1 -> Out1/1
  Integrator1/1 -> Ws->kWh/1
  In1/1 -> Integrator1/1

== system building_EXAMPLE_v1/DATALOGGER/logger_BDB/z7/Subsystem3 ==
  In1 : Inport
  Integrator1 : Integrator
  Ws->kWh : Gain  Gain=1/3600/1000
  Out1 : Outport
  wires:
  In1/1 -> Integrator1/1
  Integrator1/1 -> Ws->kWh/1
  Ws->kWh/1 -> Out1/1

== system building_EXAMPLE_v1/DATALOGGER/logger_BDB/z7/Subsystem4 ==
  In1 : Inport
  Integrator1 : Integrator
  Ws->kWh : Gain  Gain=1/3600/1000
  Out1 : Outport
  wires:
  Ws->kWh/1 -> Out1/1
  Integrator1/1 -> Ws->kWh/1
  In1/1 -> Integrator1/1

== system building_EXAMPLE_v1/DATALOGGER/logger_BDB/z7/Subsystem5 ==
  In1 : Inport
  Integrator1 : Integrator
  Ws->kWh : Gain  Gain=1/3600/1000
  Out1 : Outport
  wires:
  In1/1 -> Integrator1/1
  Integrator1/1 -> Ws->kWh/1
  Ws->kWh/1 -> Out1/1

== system building_EXAMPLE_v1/DATALOGGER/logger_BDB/z7/Subsystem6 ==
  In1 : Inport
  Integrator1 : Integrator
  Ws->kWh : Gain  Gain=1/3600/1000
  Out1 : Outport
  wires:
  Ws->kWh/1 -> Out1/1
  Integrator1/1 -> Ws->kWh/1
  In1/1 -> Integrator1/1

== system building_EXAMPLE_v1/DATALOGGER/logger_BDB/z7/Subsystem7 ==
  In1 : Inport
  Integrator1 : Integrator
  Ws->kWh : Gain  Gain=1/3600/1000
  Out1 : Outport
  wires:
  In1/1 -> Integrator1/1
  Integrator1/1 -> Ws->kWh/1
  Ws->kWh/1 -> Out1/1

== system building_EXAMPLE_v1/DATALOGGER/logger_BDB/z7/Subsystem8 ==
  In1 : Inport
  Integrator1 : Integrator
  Ws->kWh : Gain  Gain=1/3600/1000
  Out1 : Outport
  wires:
  Ws->kWh/1 -> Out1/1
  Integrator1/1 -> Ws->kWh/1
  In1/1 -> Integrator1/1

== system building_EXAMPLE_v1/DATALOGGER/logger_BDB/z7/Subsystem9 ==
  In1 : Inport
  Integrator1 : Integrator
  Ws->kWh : Gain  Gain=1/3600/1000
  Out1 : Outport
  wires:
  In1/1 -> Integrator1/1
  Integrator1/1 -> Ws->kWh/1
  Ws->kWh/1 -> Out1/1

== system building_EXAMPLE_v1/DATALOGGER/logger_BDB/z8/Subsystem ==
  In1 : Inport
  Integrator1 : Integrator
  Ws->kWh : Gain  Gain=1/3600/1000
  Out1 : Outport
  wires:
  In1/1 -> Integrator1/1
  Integrator1/1 -> Ws->kWh/1
  Ws->kWh/1 -> Out1/1

== system building_EXAMPLE_v1/DATALOGGER/logger_BDB/z8/Subsystem1 ==
  In1 : Inport
  Integrator1 : Integrator
  Ws->kWh : Gain  Gain=1/3600/1000
  Out1 : Outport
  wires:
  Ws->kWh/1 -> Out1/1
  Integrator1/1 -> Ws->kWh/1
  In1/1 -> Integrator1/1

== system building_EXAMPLE_v1/DATALOGGER/logger_BDB/z8/Subsystem10 ==
  In1 : Inport
  Integrator1 : Integrator
  Ws->kWh : Gain  Gain=1/3600/1000
  Out1 : Outport
  wires:
  In1/1 -> Integrator1/1
  Integrator1/1 -> Ws->kWh/1
  Ws->kWh/1 -> Out1/1

== system building_EXAMPLE_v1/DATALOGGER/logger_BDB/z8/Subsystem11 ==
  In1 : Inport
  Integrator1 : Integrator
  Ws->kWh : Gain  Gain=1/3600/1000
  Out1 : Outport
  wires:
  Ws->kWh/1 -> Out1/1
  Integrator1/1 -> Ws->kWh/1
  In1/1 -> Integrator1/1

== system building_EXAMPLE_v1/DATALOGGER/logger_BDB/z8/Subsystem12 ==
  In1 : Inport
  Integrator1 : Integrator
  Ws->kWh : Gain  Gain=1/3600/1000
  Out1 : Outport
  wires:
  In1/1 -> Integrator1/1
  Integrator1/1 -> Ws->kWh/1
  Ws->kWh/1 -> Out1/1

== system building_EXAMPLE_v1/DATALOGGER/logger_BDB/z8/Subsystem2 ==
  In1 : Inport
  Integrator1 : Integrator
  Ws->kWh : Gain  Gain=1/3600/1000
  Out1 : Outport
  wires:
  In1/1 -> Integrator1/1
  Integrator1/1 -> Ws->kWh/1
  Ws->kWh/1 -> Out1/1

== system building_EXAMPLE_v1/DATALOGGER/logger_BDB/z8/Subsystem3 ==
  In1 : Inport
  Integrator1 : Integrator
  Ws->kWh : Gain  Gain=1/3600/1000
  Out1 : Outport
  wires:
  Ws->kWh/1 -> Out1/1
  Integrator1/1 -> Ws->kWh/1
  In1/1 -> Integrator1/1

== system building_EXAMPLE_v1/DATALOGGER/logger_BDB/z8/Subsystem4 ==
  In1 : Inport
  Integrator1 : Integrator
  Ws->kWh : Gain  Gain=1/3600/1000
  Out1 : Outport
  wires:
  In1/1 -> Integrator1/1
  Integrator1/1 -> Ws->kWh/1
  Ws->kWh/1 -> Out1/1

== system building_EXAMPLE_v1/DATALOGGER/logger_BDB/z8/Subsystem5 ==
  In1 : Inport
  Integrator1 : Integrator
  Ws->kWh : Gain  Gain=1/3600/1000
  Out1 : Outport
  wires:
  Ws->kWh/1 -> Out1/1
  Integrator1/1 -> Ws->kWh/1
  In1/1 -> Integrator1/1

== system building_EXAMPLE_v1/DATALOGGER/logger_BDB/z8/Subsystem6 ==
  In1 : Inport
  Integrator1 : Integrator
  Ws->kWh : Gain  Gain=1/3600/1000
  Out1 : Outport
  wires:
  In1/1 -> Integrator1/1
  Integrator1/1 -> Ws->kWh/1
  Ws->kWh/1 -> Out1/1

== system building_EXAMPLE_v1/DATALOGGER/logger_BDB/z8/Subsystem7 ==
  In1 : Inport
  Integrator1 : Integrator
  Ws->kWh : Gain  Gain=1/3600/1000
  Out1 : Outport
  wires:
  Ws->kWh/1 -> Out1/1
  Integrator1/1 -> Ws->kWh/1
  In1/1 -> Integrator1/1

== system building_EXAMPLE_v1/DATALOGGER/logger_BDB/z8/Subsystem8 ==
  In1 : Inport
  Integrator1 : Integrator
  Ws->kWh : Gain  Gain=1/3600/1000
  Out1 : Outport
  wires:
  In1/1 -> Integrator1/1
  Integrator1/1 -> Ws->kWh/1
  Ws->kWh/1 -> Out1/1

== system building_EXAMPLE_v1/DATALOGGER/logger_BDB/z8/Subsystem9 ==
  In1 : Inport
  Integrator1 : Integrator
  Ws->kWh : Gain  Gain=1/3600/1000
  Out1 : Outport
  wires:
  Ws->kWh/1 -> Out1/1
  Integrator1/1 -> Ws->kWh/1
  In1/1 -> Integrator1/1

== system building_EXAMPLE_v1/DATALOGGER/logger_BDB/z9/Subsystem ==
  In1 : Inport
  Integrator1 : Integrator
  Ws->kWh : Gain  Gain=1/3600/1000
  Out1 : Outport
  wires:
  Ws->kWh/1 -> Out1/1
  Integrator1/1 -> Ws->kWh/1
  In1/1 -> Integrator1/1

== system building_EXAMPLE_v1/DATALOGGER/logger_BDB/z9/Subsystem1 ==
  In1 : Inport
  Integrator1 : Integrator
  Ws->kWh : Gain  Gain=1/3600/1000
  Out1 : Outport
  wires:
  In1/1 -> Integrator1/1
  Integrator1/1 -> Ws->kWh/1
  Ws->kWh/1 -> Out1/1

== system building_EXAMPLE_v1/DATALOGGER/logger_BDB/z9/Subsystem10 ==
  In1 : Inport
  Integrator1 : Integrator
  Ws->kWh : Gain  Gain=1/3600/1000
  Out1 : Outport
  wires:
  Ws->kWh/1 -> Out1/1
  Integrator1/1 -> Ws->kWh/1
  In1/1 -> Integrator1/1

== system building_EXAMPLE_v1/DATALOGGER/logger_BDB/z9/Subsystem11 ==
  In1 : Inport
  Integrator1 : Integrator
  Ws->kWh : Gain  Gain=1/3600/1000
  Out1 : Outport
  wires:
  In1/1 -> Integrator1/1
  Integrator1/1 -> Ws->kWh/1
  Ws->kWh/1 -> Out1/1

== system building_EXAMPLE_v1/DATALOGGER/logger_BDB/z9/Subsystem12 ==
  In1 : Inport
  Integrator1 : Integrator
  Ws->kWh : Gain  Gain=1/3600/1000
  Out1 : Outport
  wires:
  Ws->kWh/1 -> Out1/1
  Integrator1/1 -> Ws->kWh/1
  In1/1 -> Integrator1/1

== system building_EXAMPLE_v1/DATALOGGER/logger_BDB/z9/Subsystem2 ==
  In1 : Inport
  Integrator1 : Integrator
  Ws->kWh : Gain  Gain=1/3600/1000
  Out1 : Outport
  wires:
  Ws->kWh/1 -> Out1/1
  Integrator1/1 -> Ws->kWh/1
  In1/1 -> Integrator1/1

== system building_EXAMPLE_v1/DATALOGGER/logger_BDB/z9/Subsystem3 ==
  In1 : Inport
  Integrator1 : Integrator
  Ws->kWh : Gain  Gain=1/3600/1000
  Out1 : Outport
  wires:
  In1/1 -> Integrator1/1
  Integrator1/1 -> Ws->kWh/1
  Ws->kWh/1 -> Out1/1

== system building_EXAMPLE_v1/DATALOGGER/logger_BDB/z9/Subsystem4 ==
  In1 : Inport
  Integrator1 : Integrator
  Ws->kWh : Gain  Gain=1/3600/1000
  Out1 : Outport
  wires:
  Ws->kWh/1 -> Out1/1
  Integrator1/1 -> Ws->kWh/1
  In1/1 -> Integrator1/1

== system building_EXAMPLE_v1/DATALOGGER/logger_BDB/z9/Subsystem5 ==
  In1 : Inport
  Integrator1 : Integrator
  Ws->kWh : Gain  Gain=1/3600/1000
  Out1 : Outport
  wires:
  In1/1 -> Integrator1/1
  Integrator1/1 -> Ws->kWh/1
  Ws->kWh/1 -> Out1/1

== system building_EXAMPLE_v1/DATALOGGER/logger_BDB/z9/Subsystem6 ==
  In1 : Inport
  Integrator1 : Integrator
  Ws->kWh : Gain  Gain=1/3600/1000
  Out1 : Outport
  wires:
  Ws->kWh/1 -> Out1/1
  Integrator1/1 -> Ws->kWh/1
  In1/1 -> Integrator1/1

== system building_EXAMPLE_v1/DATALOGGER/logger_BDB/z9/Subsystem7 ==
  In1 : Inport
  Integrator1 : Integrator
  Ws->kWh : Gain  Gain=1/3600/1000
  Out1 : Outport
  wires:
  In1/1 -> Integrator1/1
  Integrator1/1 -> Ws->kWh/1
  Ws->kWh/1 -> Out1/1

== system building_EXAMPLE_v1/DATALOGGER/logger_BDB/z9/Subsystem8 ==
  In1 : Inport
  Integrator1 : Integrator
  Ws->kWh : Gain  Gain=1/3600/1000
  Out1 : Outport
  wires:
  Ws->kWh/1 -> Out1/1
  Integrator1/1 -> Ws->kWh/1
  In1/1 -> Integrator1/1

== system building_EXAMPLE_v1/DATALOGGER/logger_BDB/z9/Subsystem9 ==
  In1 : Inport
  Integrator1 : Integrator
  Ws->kWh : Gain  Gain=1/3600/1000
  Out1 : Outport
  wires:
  In1/1 -> Integrator1/1
  Integrator1/1 -> Ws->kWh/1
  Ws->kWh/1 -> Out1/1

== system building_EXAMPLE_v1/HVAC pipes/Pipes_outlet/Subsystem/supply ==
  T : Inport
  mdot : Inport  Port=2
  p : Inport  Port=3
  mix : Inport  Port=4
  Ground : Ground
  Mux1 : Mux  Inputs=[1 1 1 1 1 1 1 13]
  const : Constant
  const2 : Constant  Value=fluid
  const4 : Constant  Value=dia
  THV : Outport  InitialOutput=0
  wires:
  const4/1 -> Mux1/7
  mix/1 -> Mux1/6
  const2/1 -> Mux1/5
  Ground/1 -> Mux1/8
  Mux1/1 -> THV/1
  const/1 -> Mux1/1
  T/1 -> Mux1/2
  mdot/1 -> Mux1/3
  p/1 -> Mux1/4

== system building_EXAMPLE_v1/HVAC pipes/Pipes_outlet/Subsystem/supply1 ==
  T : Inport
  mdot : Inport  Port=2
  p : Inport  Port=3
  mix : Inport  Port=4
  Ground : Ground
  Mux1 : Mux  Inputs=[1 1 1 1 1 1 1 13]
  const : Constant
  const2 : Constant  Value=fluid
  const4 : Constant  Value=dia
  THV : Outport  InitialOutput=0
  wires:
  const4/1 -> Mux1/7
  mix/1 -> Mux1/6
  const2/1 -> Mux1/5
  Ground/1 -> Mux1/8
  Mux1/1 -> THV/1
  const/1 -> Mux1/1
  T/1 -> Mux1/2
  mdot/1 -> Mux1/3
  p/1 -> Mux1/4

== system building_EXAMPLE_v1/HVAC pipes/ventilation_outlet1_z1/create_THB/THB_set_mix ==
  THB_in : Inport
  mix : Inport  Port=2
  Bus Assignment : BusAssignment  AssignedSignals=FluidMix
  THB : Outport
  wires:
  THB_in/1 -> Bus Assignment/1
  Bus Assignment/1 -> THB/1
  mix/1 -> Bus Assignment/2

== system building_EXAMPLE_v1/HVAC pipes/ventilation_outlet1_z1/create_THB/THB_set_p ==
  THB_in : Inport
  p : Inport  Port=2
  Bus Assignment : BusAssignment  AssignedSignals=Pressure
  THB : Outport
  wires:
  p/1 -> Bus Assignment/2
  Bus Assignment/1 -> THB/1
  THB_in/1 -> Bus Assignment/1

== system building_EXAMPLE_v1/HVAC pipes/ventilation_outlet1_z10/create_THB/THB_set_mix ==
  THB_in : Inport
  mix : Inport  Port=2
  Bus Assignment : BusAssignment  AssignedSignals=FluidMix
  THB : Outport
  wires:
  THB_in/1 -> Bus Assignment/1
  Bus Assignment/1 -> THB/1
  mix/1 -> Bus Assignment/2

== system building_EXAMPLE_v1/HVAC pipes/ventilation_outlet1_z10/create_THB/THB_set_p ==
  THB_in : Inport
  p : Inport  Port=2
  Bus Assignment : BusAssignment  AssignedSignals=Pressure
  THB : Outport
  wires:
  p/1 -> Bus Assignment/2
  Bus Assignment/1 -> THB/1
  THB_in/1 -> Bus Assignment/1

== system building_EXAMPLE_v1/HVAC pipes/ventilation_outlet1_z2/create_THB/THB_set_mix ==
  THB_in : Inport
  mix : Inport  Port=2
  Bus Assignment : BusAssignment  AssignedSignals=FluidMix
  THB : Outport
  wires:
  THB_in/1 -> Bus Assignment/1
  Bus Assignment/1 -> THB/1
  mix/1 -> Bus Assignment/2

== system building_EXAMPLE_v1/HVAC pipes/ventilation_outlet1_z2/create_THB/THB_set_p ==
  THB_in : Inport
  p : Inport  Port=2
  Bus Assignment : BusAssignment  AssignedSignals=Pressure
  THB : Outport
  wires:
  p/1 -> Bus Assignment/2
  Bus Assignment/1 -> THB/1
  THB_in/1 -> Bus Assignment/1

== system building_EXAMPLE_v1/HVAC pipes/ventilation_outlet1_z3/create_THB/THB_set_mix ==
  THB_in : Inport
  mix : Inport  Port=2
  Bus Assignment : BusAssignment  AssignedSignals=FluidMix
  THB : Outport
  wires:
  THB_in/1 -> Bus Assignment/1
  Bus Assignment/1 -> THB/1
  mix/1 -> Bus Assignment/2

== system building_EXAMPLE_v1/HVAC pipes/ventilation_outlet1_z3/create_THB/THB_set_p ==
  THB_in : Inport
  p : Inport  Port=2
  Bus Assignment : BusAssignment  AssignedSignals=Pressure
  THB : Outport
  wires:
  p/1 -> Bus Assignment/2
  Bus Assignment/1 -> THB/1
  THB_in/1 -> Bus Assignment/1

== system building_EXAMPLE_v1/HVAC pipes/ventilation_outlet1_z4/create_THB/THB_set_mix ==
  THB_in : Inport
  mix : Inport  Port=2
  Bus Assignment : BusAssignment  AssignedSignals=FluidMix
  THB : Outport
  wires:
  THB_in/1 -> Bus Assignment/1
  Bus Assignment/1 -> THB/1
  mix/1 -> Bus Assignment/2

== system building_EXAMPLE_v1/HVAC pipes/ventilation_outlet1_z4/create_THB/THB_set_p ==
  THB_in : Inport
  p : Inport  Port=2
  Bus Assignment : BusAssignment  AssignedSignals=Pressure
  THB : Outport
  wires:
  p/1 -> Bus Assignment/2
  Bus Assignment/1 -> THB/1
  THB_in/1 -> Bus Assignment/1

== system building_EXAMPLE_v1/HVAC pipes/ventilation_outlet1_z5/create_THB/THB_set_mix ==
  THB_in : Inport
  mix : Inport  Port=2
  Bus Assignment : BusAssignment  AssignedSignals=FluidMix
  THB : Outport
  wires:
  THB_in/1 -> Bus Assignment/1
  Bus Assignment/1 -> THB/1
  mix/1 -> Bus Assignment/2

== system building_EXAMPLE_v1/HVAC pipes/ventilation_outlet1_z5/create_THB/THB_set_p ==
  THB_in : Inport
  p : Inport  Port=2
  Bus Assignment : BusAssignment  AssignedSignals=Pressure
  THB : Outport
  wires:
  p/1 -> Bus Assignment/2
  Bus Assignment/1 -> THB/1
  THB_in/1 -> Bus Assignment/1

== system building_EXAMPLE_v1/HVAC pipes/ventilation_outlet1_z6/create_THB/THB_set_mix ==
  THB_in : Inport
  mix : Inport  Port=2
  Bus Assignment : BusAssignment  AssignedSignals=FluidMix
  THB : Outport
  wires:
  THB_in/1 -> Bus Assignment/1
  Bus Assignment/1 -> THB/1
  mix/1 -> Bus Assignment/2

== system building_EXAMPLE_v1/HVAC pipes/ventilation_outlet1_z6/create_THB/THB_set_p ==
  THB_in : Inport
  p : Inport  Port=2
  Bus Assignment : BusAssignment  AssignedSignals=Pressure
  THB : Outport
  wires:
  p/1 -> Bus Assignment/2
  Bus Assignment/1 -> THB/1
  THB_in/1 -> Bus Assignment/1

== system building_EXAMPLE_v1/HVAC pipes/ventilation_outlet1_z7/create_THB/THB_set_mix ==
  THB_in : Inport
  mix : Inport  Port=2
  Bus Assignment : BusAssignment  AssignedSignals=FluidMix
  THB : Outport
  wires:
  THB_in/1 -> Bus Assignment/1
  Bus Assignment/1 -> THB/1
  mix/1 -> Bus Assignment/2

== system building_EXAMPLE_v1/HVAC pipes/ventilation_outlet1_z7/create_THB/THB_set_p ==
  THB_in : Inport
  p : Inport  Port=2
  Bus Assignment : BusAssignment  AssignedSignals=Pressure
  THB : Outport
  wires:
  p/1 -> Bus Assignment/2
  Bus Assignment/1 -> THB/1
  THB_in/1 -> Bus Assignment/1

== system building_EXAMPLE_v1/HVAC pipes/ventilation_outlet1_z8/create_THB/THB_set_mix ==
  THB_in : Inport
  mix : Inport  Port=2
  Bus Assignment : BusAssignment  AssignedSignals=FluidMix
  THB : Outport
  wires:
  THB_in/1 -> Bus Assignment/1
  Bus Assignment/1 -> THB/1
  mix/1 -> Bus Assignment/2

== system building_EXAMPLE_v1/HVAC pipes/ventilation_outlet1_z8/create_THB/THB_set_p ==
  THB_in : Inport
  p : Inport  Port=2
  Bus Assignment : BusAssignment  AssignedSignals=Pressure
  THB : Outport
  wires:
  p/1 -> Bus Assignment/2
  Bus Assignment/1 -> THB/1
  THB_in/1 -> Bus Assignment/1

== system building_EXAMPLE_v1/HVAC pipes/ventilation_outlet1_z9/create_THB/THB_set_mix ==
  THB_in : Inport
  mix : Inport  Port=2
  Bus Assignment : BusAssignment  AssignedSignals=FluidMix
  THB : Outport
  wires:
  THB_in/1 -> Bus Assignment/1
  Bus Assignment/1 -> THB/1
  mix/1 -> Bus Assignment/2

== system building_EXAMPLE_v1/HVAC pipes/ventilation_outlet1_z9/create_THB/THB_set_p ==
  THB_in : Inport
  p : Inport  Port=2
  Bus Assignment : BusAssignment  AssignedSignals=Pressure
  THB : Outport
  wires:
  p/1 -> Bus Assignment/2
  Bus Assignment/1 -> THB/1
  THB_in/1 -> Bus Assignment/1
